simulink model "singledof_base"  (Simulink 7.8)
settings: Solver=FixedStepDiscrete  StartTime=0.0  StopTime=inf  FixedStep=Ts  RelTol=1e-3
PreLoadFcn:
  | loadParametersSingleDof
InitFcn:
  | loadParametersSingleDof
values from neighbouring files (symbols this model uses):
  L_arm = 0.075    [freemot.mat]    (also in loadParametersSingleDof.m)
  lowOrder_tfd_foh = c2d(tf([1 2*pi*.64154],[1 0]),Ts,'foh')    [loadParametersSingleDof.m]
  maxTorque_allowed = 1.125    [freemot.mat]    (also in loadParametersSingleDof.m)
  torque_constant = 3.112    [freemot.mat]    (also in loadParametersSingleDof.m)
  Ts = 0.0005    [freemot.mat]
undefined symbols (not defined in the file or in its folder): DiscIntNeverNeededParam, shuntDynPredict_part1_tfd_foh, shuntDynPredict_part2_tfd_foh
libraries: simulink x30, simulink_extras x3
(part 1 of 2)
settings Model: Creator=root  LastModifiedBy=root  SimulationMode=external  ExtModeTrigDuration=10000  ExtModeAutoUpdateStatusClock=off
settings OptimizationCC: InitFltsAndDblsToZero=on
settings DebuggingCC: SaveWithParameterizedLinksMsg=none  SignalResolutionControl=TryResolveAllWithWarning  MultiTaskDSMMsg=warning  MultiTaskCondExecSysMsg=none  FcnCallInpInsideContextMsg=Use local settings  StrictBusMsg=None
settings RTWCC: SystemTargetFile=ectarget.tlc  MakeCommand=make_rtw OPTS='-DNETIF_ID=1'  TemplateMakefile=ec_unix.tmf  Description=Ethercattarget Real-Time Target for PREEMPT-RT/Linux  ProcessScript=ectarget_make_rtw_hook  IncludeERTFirstTime=on
settings GRTTargetCC: TargetFcnLib=ansi_tfl_tmw.mat  ExtMode=on

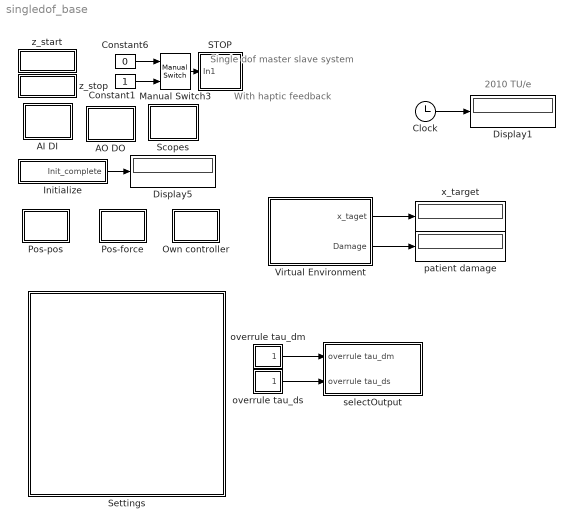
== system singledof_base ==
  note: With haptic feedback
  note: 2010 TU/e
  note: Single dof master slave system
  AI DI : Subsystem
      mask Display: disp('AI / DI')
  AO DO : Subsystem
      mask Display: disp('AO / DO')
  Clock : Clock
  Constant1 : Constant
  Constant6 : Constant  Value=0
  Display1 : Display
      settings: Decimation=200
  Display5 : Display
      settings: Decimation=200
  Initialize : Subsystem
  Manual Switch3 : simulink/Signal Routing/Manual Switch  sw=1  action=0  varsize=off
  Own controller : Subsystem
  Pos-force : Subsystem  mask{Ps=8, Is=0, Ds=0.1, bw_mode=off, fc=20, useI=on}
      mask prompts: Ps "Proportional action Position Slave"; Is "Integral action Position Slave"; Ds "Differential action Position Slave"; bw_mode "Or enter bandwidth:"; fc "Enter bandwidth (Hz) (max 70Hz)"; useI "Use Integral action"
      mask CallbackString:
      | |||temp=get_param(gcb,'bw_mode');
      | 
      | if(strcmp(temp,'off'))
      |    set_param(gcb,'MaskEnables',{'on','on','on','on','off','off'})
      | else
      |        set_param(gcb,'MaskEnables',{'off','off','off','on','on','on'})
      | end|
      | if strcmp(get_param(gcb,'bw_mode'),'on')
      |     wc=2*pi*eval(get_param(gcb,'fc'));
      |     if strcmp(get_param(gcb,'useI'),'on')
      |         C_tf=tf([1/wc 1 wc/5],[1 0]);
      |     else
      |         C_tf=tf([1/wc 1],1);
      |     end
      |     C_tf=minreal(C_tf/abs(freqresp(C_tf*fit_g22_s_2,wc)));
      |     set_param(gcb,'Ds',num2str(C_tf.num{1}(1)));
      |     set_param(gcb,'Ps',num2str(C_tf.num{1}(2)));
      | 
      |     if strcmp(get_param(gcb,'useI'),'on')
      |         set_param(gcb,'Is',num2str(C_tf.num{1}(3)));
      |     else
      |         set_param(gcb,'Is','0');
      |     end
      | end|temp=get_param(gcb,'maskCallbacks');
      | eval(temp{5})
  Pos-pos : Subsystem  mask{Pm=15, Im=0, Dm=.1, bw_modem=off, fcm=20, useIm=off, Ps=15, Is=0, Ds=.1, bw_modes=off, fcs=20, useIs=off}
      mask prompts: Pm "Proportional action master"; Im "Integral action master"; Dm "Differential action master"; bw_modem "Or enter bandwidth"; fcm "Bandwidth (Hz) (max 70Hz)"; useIm "Use Integral action"; Ps "Proportional action slave"; Is "Integral action slave"; Ds "Differential action slave"; bw_modes "Or enter bandwidth"; fcs "Bandwidth (Hz) (max 70Hz)"; useIs "Use Integral action"
      mask CallbackString:
      | |||temp=get_param(gcb,'bw_modem');
      | temps=get_param(gcb,'bw_modes');
      | 
      | if strcmp(temp,'off') & strcmp(temps,'off')
      |    set_param(gcb,'MaskEnables',{'on','on','on','on','off','off','on','on','on','on','off','off'})
      | elseif strcmp(temp,'on') & strcmp(temps,'off')
      |    set_param(gcb,'MaskEnables',{'off','off','off','on','on','on','on','on','on','on','off','off'})
      | elseif strcmp(temp,'off') & strcmp(temps,'on')
      |    set_param(gcb,'MaskEnables',{'on','on','on','on','off','off','off','off','off','on','on','on'})
      | else
      |    set_param(gcb,'MaskEnables',{'off','off','off','on','on','on','off','off','off','on','on','on'})
      | end|if strcmp(get_param(gcb,'bw_modem'),'on')
      |     wc=2*pi*eval(get_param(gcb,'fcm'));
      |     if strcmp(get_param(gcb,'useIm'),'on')
      |         C_tf=tf([1/wc 1 wc/5],[1 0]);
      |     else
      |         C_tf=tf([1/wc 1],1);
      |     end
      |     C_tf=minreal(C_tf/abs(freqresp(C_tf*fit_g22_m_2,wc)));
      |     set_param(gcb,'Dm',num2str(C_tf.num{1}(1)));
      |     set_param(gcb,'Pm',num2str(C_tf.num{1}(2)));
      | 
      |     if strcmp(get_param(gcb,'useIm'),'on')
      |         set_param(gcb,'Im',num2str(C_tf.num{1}(3)));
      |     else
      |         set_param(gcb,'Im','0');
      |     end
      | end|temp=get_param(gcb,'maskCallbacks');
      | eval(temp{5})||||temp=get_param(gcb,'maskCallbacks');
      | eval(temp{4})|if strcmp(get_param(gcb,'bw_modes'),'on')
      |     wc=2*pi*eval(get_param(gcb,'fcs'));
      |     if strcmp(get_param(gcb,'useIs'),'on')
      |         C_tf=tf([1/wc 1 wc/5],[1 0]);
      |     else
      |         C_tf=tf([1/wc 1],1);
      |     end
      |     C_tf=minreal(C_tf/abs(freqresp(C_tf*fit_g22_s_2,wc)));
      |     set_param(gcb,'Ds',num2str(C_tf.num{1}(1)));
      |     set_param(gcb,'Ps',num2str(C_tf.num{1}(2)));
      | 
      |     if strcmp(get_param(gcb,'useIs'),'on')
      |         set_param(gcb,'Is',num2str(C_tf.num{1}(3)));
      |     else
      |         set_param(gcb,'Is','0');
      |     end
      | end|temp=get_param(gcb,'maskCallbacks');
      | eval(temp{11})
  STOP : Subsystem
  Scopes : Subsystem
      mask Display: disp('Scopes')
  Settings : Subsystem  mask{mode=Own-controller, mu=1, lambda=1, comm_delay=0}
      mask prompts: mode "Control algorithm"; mu "Position scaling (mu)"; lambda "Force scaling (lambda)"; comm_delay "Communication delay"
      mask init:
      | bn{1}='off';
      | bn{2}='on';
      mask StyleString: popup(Position-position|Position-force|Own-controller|Overrule),edit,edit,edit
      mask Display:
      | text(.05,15/16,['Active mode: ' get_param(gcb,'mode')])
      | 
      | text(.05,13/16,['Position scaling (mu): ' num2str(mu)])
      | text(.05,12/16,['Force scaling (lambda): ' num2str(lambda)])
      | 
      | text(.05,10/16,['Communication delay: ' num2str(comm_delay) ' s'])
  Virtual Environment : Subsystem
  overrule tau_dm : Subsystem  LoadFcn=slideg Load  StartFcn=slideg StartFcn  StopFcn=slideg StopFcn  mask(Slider Gain){low=0, gain=0, high=0.5}
      settings: CopyFcn=slideg Copy  DeleteFcn=slideg DeleteBlock  NameChangeFcn=slideg NameChange  OpenFcn=slideg Open  CloseFcn=slideg Close  ParentCloseFcn=slideg ParentClose
      mask Display: disp(gain)
  overrule tau_ds : Subsystem  LoadFcn=slideg Load  StartFcn=slideg StartFcn  StopFcn=slideg StopFcn  mask(Slider Gain){low=0, gain=0, high=0.5}
      settings: CopyFcn=slideg Copy  DeleteFcn=slideg DeleteBlock  NameChangeFcn=slideg NameChange  OpenFcn=slideg Open  CloseFcn=slideg Close  ParentCloseFcn=slideg ParentClose
      mask Display: disp(gain)
  patient damage : Display
  selectOutput : Subsystem
  x_target : Display
  z_start : Subsystem
      settings: OpenFcn=|
      | set_param(bdroot(gcs),'SimulationCommand','connect')
      | set_param(bdroot(gcs),'SimulationCommand','start')
      mask Display: disp('start')
  z_stop : Subsystem
      settings: OpenFcn=set_param('singledof_demo/Initialize/ShutdownSim','Value',int2str(eval(get_param('singledof_demo/Initialize/ShutdownSim','Value'))+1))
      mask Display: disp('stop')
  wires:
  Initialize/1(Init_complete) -> Display5/1
  Clock/1 -> Display1/1
  Manual Switch3/1 -> STOP/1(In1)
  Constant6/1 -> Manual Switch3/1
  Constant1/1 -> Manual Switch3/2
  overrule tau_dm/1(Out1) -> selectOutput/1(overrule tau_dm)
  overrule tau_ds/1(Out1) -> selectOutput/2(overrule tau_ds)
  Virtual Environment/1(x_taget) -> x_target/1
  Virtual Environment/2(Damage) -> patient damage/1

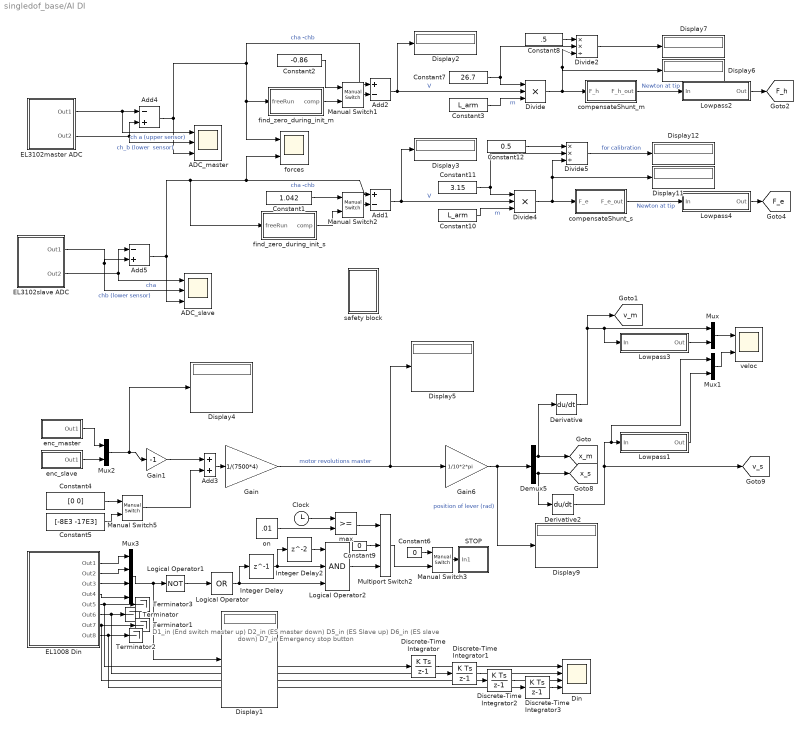
== system singledof_base/AI DI ==
  note: D1_in (End switch master up)
      | D2_in (ES master down)
      | D5_in (ES Slave up)
      | D6_in (ES slave down)
      | D7_in Emergency stop button
  ADC_master : Scope  NumInputPorts=3
      settings: TimeRange=5  YMin=7.605~1.4075~-6.204  YMax=7.6275~1.43~-6.192  SaveName=env_est2  MaxDataPoints=10000
  ADC_slave : Scope  NumInputPorts=3
      settings: TimeRange=5  YMin=2.775~-5~-7.5  YMax=2.975~10~7.5  SaveName=env_est3  MaxDataPoints=10000
  Add1 : Sum  Inputs=+-
  Add2 : Sum  Inputs=+-
  Add3 : Sum
  Add4 : Sum  Inputs=-+
  Add5 : Sum  Inputs=-+
  Clock : Clock
  Constant1 : Constant  Value=1.042
  Constant10 : Constant  Value=L_arm
  Constant11 : Constant  Value=3.15
  Constant12 : Constant  Value=0.5
  Constant2 : Constant  Value=-0.86
  Constant3 : Constant  Value=L_arm
  Constant4 : Constant  Value=[0 0]
  Constant5 : Constant  Value=[-8E3 -17E3]
  Constant6 : Constant  Value=0
  Constant7 : Constant  Value=26.7
  Constant8 : Constant  Value=.5
  Constant9 : Constant  Value=0
  Demux5 : Demux  Outputs=2
  Derivative : Derivative
  Derivative2 : Derivative
  Din : Scope  NumInputPorts=4
      settings: TimeRange=5  YMin=-5~-5~-5~-5  YMax=10~10~5~5  SaveName=env_est5  MaxDataPoints=10000
  Discrete-Time Integrator{,1..3} (4 alike) : DiscreteIntegrator  SampleTime=Ts  ICPrevOutput=DiscIntNeverNeededParam  ICPrevScaledInput=DiscIntNeverNeededParam
  Display{1..7,9,11..12} (10 alike) : Display
      settings: Decimation=200
  Divide : Product  Inputs=***
  Divide2 : Product  Inputs=**/
  Divide4 : Product  Inputs=***
  Divide5 : Product  Inputs=**/
  EL1008 Din : Subsystem  mask(EL1008){link_id=0}
      mask prompts: link_id "Link id (>=0)"
  EL3102master ADC : Subsystem  mask(EL3102){link_id=0}
      mask prompts: link_id "Link id (>=0)"
  EL3102slave ADC : Subsystem  mask(EL3102){link_id=1}
      mask prompts: link_id "Link id (>=0)"
  Gain : Gain  Gain=1/(7500*4)
  Gain1 : Gain  Gain=-1
  Gain6 : Gain  Gain=1/10*2*pi
  Integer Delay : Delay  DelayLength=1
  Integer Delay2 : Delay
  Logical Operator : Logic  Operator=OR  Inputs=1  AllPortsSameDT=off  OutDataTypeStr=boolean
  Logical Operator1 : Logic  Operator=NOT  Inputs=1  AllPortsSameDT=off  OutDataTypeStr=boolean
  Logical Operator2 : Logic  Inputs=3  AllPortsSameDT=off  OutDataTypeStr=boolean
  Lowpass1 : Subsystem  mask{cf=100}
      mask prompts: cf "Cut off Frequency"
      mask help:
      | Discrete time first order lowpass filter, with cut-off frequency cf (Hz)
      | Kz / (z+K-1), with K=2*pi*cf*TS
      | For low frequencies this corresponds to the continous time lowpass filter
      | tf(1,[1/(2*pi*cf) 1])
      |
      | The maximum value for K=1, in this case output equals input
      | e.g. for 4000Hz sampling frequency the maximum value cf=4000/(2*pi)=637Hz.
      mask Display: text(.1,.5,['Lowpass @' num2str(cf) 'Hz'])
  Lowpass2 : Subsystem  mask{cf=40}
      mask prompts: cf "Cut off Frequency"
      mask help:
      | Discrete time first order lowpass filter, with cut-off frequency cf (Hz)
      | Kz / (z+K-1), with K=2*pi*cf*TS
      | For low frequencies this corresponds to the continous time lowpass filter
      | tf(1,[1/(2*pi*cf) 1])
      |
      | The maximum value for K=1, in this case output equals input
      | e.g. for 4000Hz sampling frequency the maximum value cf=4000/(2*pi)=637Hz.
      mask Display: text(.1,.5,['Lowpass @' num2str(cf) 'Hz'])
  Lowpass3 : Subsystem  mask{cf=100}
      mask prompts: cf "Cut off Frequency"
      mask help:
      | Discrete time first order lowpass filter, with cut-off frequency cf (Hz)
      | Kz / (z+K-1), with K=2*pi*cf*TS
      | For low frequencies this corresponds to the continous time lowpass filter
      | tf(1,[1/(2*pi*cf) 1])
      |
      | The maximum value for K=1, in this case output equals input
      | e.g. for 4000Hz sampling frequency the maximum value cf=4000/(2*pi)=637Hz.
      mask Display: text(.1,.5,['Lowpass @' num2str(cf) 'Hz'])
  Lowpass4 : Subsystem  mask{cf=40}
      mask prompts: cf "Cut off Frequency"
      mask help:
      | Discrete time first order lowpass filter, with cut-off frequency cf (Hz)
      | Kz / (z+K-1), with K=2*pi*cf*TS
      | For low frequencies this corresponds to the continous time lowpass filter
      | tf(1,[1/(2*pi*cf) 1])
      |
      | The maximum value for K=1, in this case output equals input
      | e.g. for 4000Hz sampling frequency the maximum value cf=4000/(2*pi)=637Hz.
      mask Display: text(.1,.5,['Lowpass @' num2str(cf) 'Hz'])
  Manual Switch1 : simulink/Signal Routing/Manual Switch  sw=0  action=0  varsize=off
  Manual Switch2 : simulink/Signal Routing/Manual Switch  sw=0  action=0  varsize=off
  Manual Switch3 : simulink/Signal Routing/Manual Switch  sw=1  action=0  varsize=off
  Manual Switch5 : simulink/Signal Routing/Manual Switch  sw=1  action=0  varsize=off
  Multiport Switch2 : MultiPortSwitch  DataPortOrder=Zero-based contiguous  Inputs=2  zeroidx=on
  Mux : Mux  Inputs=2
  Mux1 : Mux  Inputs=2
  Mux2 : Mux  Inputs=2
  Mux3 : Mux
  STOP : Subsystem
  Terminator{,1..3} (4 alike) : Terminator
  compensateShunt_m : Subsystem
  compensateShunt_s : Subsystem
  enc_master : Subsystem
  enc_slave : Subsystem
  find_zero_during_init_m : Subsystem
  find_zero_during_init_s : Subsystem
  forces : Scope  NumInputPorts=2
      settings: TimeRange=6.25  YMin=-1.275~7.5  YMax=-0.95~9.4  SaveName=env_est4  MaxDataPoints=10000
  max : RelationalOperator  DisableCoverage=on
  on : Constant  DisableCoverage=on  Value=.01
  safety block : Subsystem
  veloc : Scope  NumInputPorts=2
      settings: TimeRange=6.25  YMin=-40000~-40000  YMax=40000~40000  SaveName=env_est1  MaxDataPoints=10000
  tag scope: F_e=global, F_h=global, v_m=global, v_s=global, x_m=global, x_s=global
  wires:
  Gain/1 -> Gain6/1, Display5/1  "motor revolutions master"
  Mux2/1 -> Gain1/1, Display4/1
  Add3/1 -> Gain/1
  Gain1/1 -> Add3/1
  Mux3/1 -> Display1/1, Logical Operator1/1
  Gain6/1 -> Demux5/1, Display9/1  "position of lever (rad)"
  Demux5/1 -> Derivative/1, [x_m]
  Demux5/2 -> Derivative2/1, [x_s]
  Derivative/1 -> Mux/1, Lowpass3/1(In), [v_m]
  Derivative2/1 -> Mux1/1, Lowpass1/1(In), [v_s]
  Logical Operator/1 -> Integer Delay/1, Logical Operator2/3
  Manual Switch3/1 -> STOP/1(In1)
  Constant6/1 -> Manual Switch3/1
  Integer Delay2/1 -> Logical Operator2/1
  Mux/1 -> veloc/1
  Mux1/1 -> veloc/2
  Lowpass3/1(Out) -> Mux/2
  Lowpass1/1(Out) -> Mux1/2
  EL1008 Din/1(Out1) -> Mux3/1
  EL1008 Din/2(Out2) -> Mux3/2
  EL1008 Din/3(Out3) -> Mux3/3
  EL1008 Din/4(Out4) -> Mux3/4
  EL1008 Din/7(Out7) -> Terminator1/1, Discrete-Time Integrator2/1
  EL1008 Din/8(Out8) -> Terminator2/1, Discrete-Time Integrator3/1
  EL1008 Din/5(Out5) -> Terminator3/1, Discrete-Time Integrator/1
  Logical Operator1/1 -> Logical Operator/1
  Integer Delay/1 -> Integer Delay2/1, Logical Operator2/2
  Constant4/1 -> Manual Switch5/1
  Constant5/1 -> Manual Switch5/2
  Manual Switch5/1 -> Add3/2
  Multiport Switch2/1 -> Manual Switch3/2
  Logical Operator2/1 -> Multiport Switch2/3
  Constant9/1 -> Multiport Switch2/2
  max/1 -> Multiport Switch2/1
  on/1 -> max/2
  Clock/1 -> max/1
  EL1008 Din/6(Out6) -> Terminator/1, Discrete-Time Integrator1/1
  Discrete-Time Integrator/1 -> Din/1
  Discrete-Time Integrator1/1 -> Din/2
  Discrete-Time Integrator2/1 -> Din/3
  Discrete-Time Integrator3/1 -> Din/4
  enc_master/1(Out1) -> Mux2/1
  enc_slave/1(Out1) -> Mux2/2
  Add2/1 -> Display2/1, Divide/2  "V"
  Manual Switch1/1 -> Add2/2
  Constant2/1 -> Manual Switch1/1
  find_zero_during_init_m/1(comp) -> Manual Switch1/2
  Divide/1 -> Display6/1, Divide2/3, compensateShunt_m/1(F_h)
  compensateShunt_m/1(F_h_out) -> Lowpass2/1(In)  "Newton at tip"
  Constant3/1 -> Divide/3  "m"
  Constant7/1 -> Divide/1, Divide2/2
  Add1/1 -> Divide4/2, Display3/1  "V"
  Manual Switch2/1 -> Add1/2
  Constant1/1 -> Manual Switch2/1
  find_zero_during_init_s/1(comp) -> Manual Switch2/2
  compensateShunt_s/1(F_e_out) -> Lowpass4/1(In)  "Newton at tip"
  Divide4/1 -> compensateShunt_s/1(F_e), Display11/1, Divide5/3
  Constant10/1 -> Divide4/3  "m"
  Constant11/1 -> Divide4/1, Divide5/2
  Constant12/1 -> Divide5/1
  Divide5/1 -> Display12/1  "for calibration"
  Lowpass2/1(Out) -> [F_h]
  Lowpass4/1(Out) -> [F_e]
  Divide2/1 -> Display7/1
  Constant8/1 -> Divide2/1
  EL3102master ADC/1(Out1) -> Add4/1, ADC_master/1  "ch a (upper sensor)"
  EL3102master ADC/2(Out2) -> ADC_master/2, Add4/2  "ch_b (lower  sensor)"
  Add4/1 -> forces/1, find_zero_during_init_m/1(freeRun), Add2/1, ADC_master/3  "cha -chb"
  EL3102slave ADC/1(Out1) -> ADC_slave/2, Add5/2  "chb (lower sensor)"
  EL3102slave ADC/2(Out2) -> ADC_slave/1, Add5/1  "cha"
  Add5/1 -> Add1/1, forces/2, find_zero_during_init_s/1(freeRun), ADC_slave/3  "cha -chb"

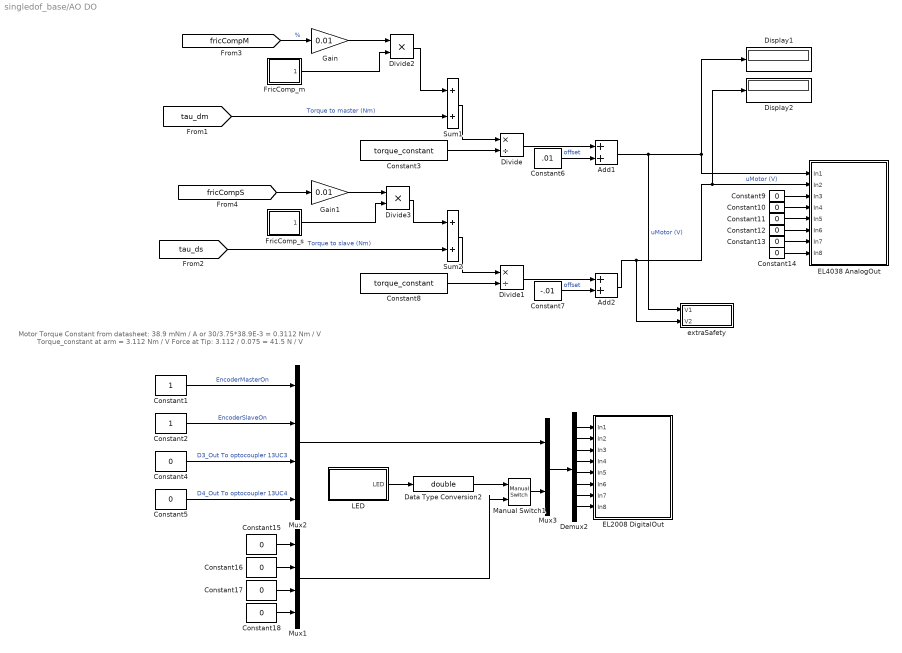
== system singledof_base/AO DO ==
  note: Motor Torque Constant from datasheet: 38.9 mNm / A or 30/3.75*38.9E-3 = 0.3112 Nm / V
      | Torque_constant at arm = 3.112 Nm / V
      | Force at Tip: 3.112 / 0.075 = 41.5 N / V
  Add1 : Sum
  Add2 : Sum
  Constant1 : Constant
  Constant{4..5,9..18} (12 alike) : Constant  Value=0
  Constant2 : Constant
  Constant3 : Constant  Value=torque_constant
  Constant6 : Constant  Value=.01
  Constant7 : Constant  Value=-.01
  Constant8 : Constant  Value=torque_constant
  Data Type Conversion2 : DataTypeConversion  OutDataTypeStr=double
  Demux2 : Demux  Outputs=8
  Display1 : Display
      settings: Decimation=200
  Display2 : Display
      settings: Decimation=200
  Divide : Product  Inputs=*/
  Divide1 : Product  Inputs=*/
  Divide2 : Product  Inputs=**
  Divide3 : Product  Inputs=**
  EL2008 DigitalOut : Subsystem  mask(EL2008){link_id=0}
      mask prompts: link_id "Link id (>=0)"
  EL4038 AnalogOut : Subsystem  mask(EL4038){link_id=0}
      mask prompts: link_id "Link id (>=0)"
  FricComp_m : Subsystem
      mask Display: plot([-1 0 0 1],[-1-2, -1, 1, 1+2], [-1 1],[0 0],[0 0],[-3,3])
  FricComp_s : Subsystem
      mask Display: plot([-1 0 0 1],[-1-2, -1, 1, 1+2], [-1 1],[0 0],[0 0],[-3,3])
  Gain : Gain  Gain=0.01
  Gain1 : Gain  Gain=0.01
  LED : Subsystem
  Manual Switch1 : simulink/Signal Routing/Manual Switch  sw=0  action=0  varsize=off
  Mux1 : Mux
  Mux2 : Mux
  Mux3 : Mux  Inputs=2
  Sum1 : Sum
  Sum2 : Sum
  extraSafety : Subsystem
  wires:
  Demux2/8 -> EL2008 DigitalOut/8(In8)
  Demux2/7 -> EL2008 DigitalOut/7(In7)
  Demux2/6 -> EL2008 DigitalOut/6(In6)
  Demux2/5 -> EL2008 DigitalOut/5(In5)
  Demux2/4 -> EL2008 DigitalOut/4(In4)
  Demux2/3 -> EL2008 DigitalOut/3(In3)
  Demux2/2 -> EL2008 DigitalOut/2(In2)
  Demux2/1 -> EL2008 DigitalOut/1(In1)
  Constant14/1 -> EL4038 AnalogOut/8(In8)
  Constant13/1 -> EL4038 AnalogOut/7(In7)
  Constant12/1 -> EL4038 AnalogOut/6(In6)
  Constant11/1 -> EL4038 AnalogOut/5(In5)
  Constant10/1 -> EL4038 AnalogOut/4(In4)
  Constant9/1 -> EL4038 AnalogOut/3(In3)
  [fricCompS] -> Gain1/1
  Gain/1 -> Divide2/1
  Divide2/1 -> Sum1/1
  Gain1/1 -> Divide3/1
  Divide3/1 -> Sum2/1
  [fricCompM] -> Gain/1  "%"
  FricComp_s/1(FricCompOut) -> Divide3/2
  FricComp_m/1(FricCompOut) -> Divide2/2
  Sum2/1 -> Divide1/1
  Sum1/1 -> Divide/1
  Mux3/1 -> Demux2/1
  LED/1(LED) -> Data Type Conversion2/1
  Mux2/1 -> Mux3/1
  [tau_ds] -> Sum2/2  "Torque to slave (Nm)"
  [tau_dm] -> Sum1/2  "Torque to master (Nm)"
  Constant8/1 -> Divide1/2
  Constant3/1 -> Divide/2
  Divide1/1 -> Add2/1
  Divide/1 -> Add1/1
  Constant7/1 -> Add2/2  "offset"
  Add2/1 -> Display2/1, EL4038 AnalogOut/2(In2), extraSafety/2(V2)  "uMotor (V)"
  Constant6/1 -> Add1/2  "offset"
  Add1/1 -> Display1/1, EL4038 AnalogOut/1(In1), extraSafety/1(V1)  "uMotor (V)"
  Constant5/1 -> Mux2/4  "D4_Out To optocoupler 13UC4"
  Constant4/1 -> Mux2/3  "D3_Out To optocoupler 13UC3"
  Constant2/1 -> Mux2/2  "EncoderSlaveOn"
  Constant1/1 -> Mux2/1  "EncoderMasterOn"
  Constant15/1 -> Mux1/1
  Constant16/1 -> Mux1/2
  Constant17/1 -> Mux1/3
  Constant18/1 -> Mux1/4
  Manual Switch1/1 -> Mux3/2
  Mux1/1 -> Manual Switch1/2
  Data Type Conversion2/1 -> Manual Switch1/1

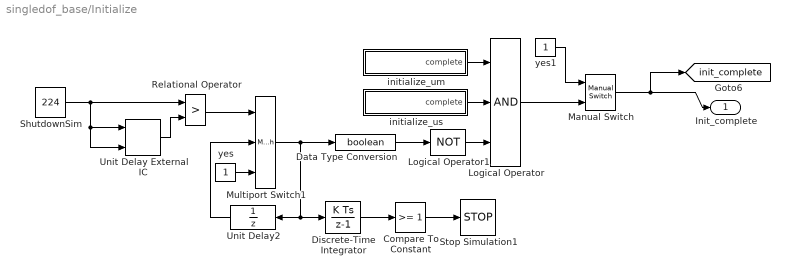
== system singledof_base/Initialize ==
  Compare To Constant : simulink/Logic and Bit Operations/Compare To Constant  relop=>=  const=1  OutDataTypeStr=boolean
  Data Type Conversion : DataTypeConversion  OutDataTypeStr=boolean
  Discrete-Time Integrator : DiscreteIntegrator  SampleTime=Ts  ICPrevOutput=DiscIntNeverNeededParam  ICPrevScaledInput=DiscIntNeverNeededParam
  Logical Operator : Logic  Inputs=3  AllPortsSameDT=off  OutDataTypeStr=boolean
  Logical Operator1 : Logic  Operator=NOT  Inputs=3  AllPortsSameDT=off  OutDataTypeStr=boolean
  Manual Switch : simulink/Signal Routing/Manual Switch  sw=1  action=0  varsize=off
  Multiport Switch1 : MultiPortSwitch  DataPortOrder=Zero-based contiguous  Inputs=2  zeroidx=on
  Relational Operator : RelationalOperator  Operator=>  OutDataTypeStr=boolean
  ShutdownSim : Constant  Value=224
  Stop Simulation1 : Stop
  Unit Delay External IC : simulink/Additional Math & Discrete/Additional Discrete/Unit Delay External IC  tsamp=-1
  Unit Delay2 : UnitDelay  SampleTime=-1
  initialize_um : Subsystem
  initialize_us : Subsystem
  yes : Constant
  yes1 : Constant
  Init_complete : Outport
  tag scope: init_complete=global
  wires:
  Manual Switch/1 -> Init_complete/1, [init_complete]
  Unit Delay External IC/1 -> Relational Operator/2
  ShutdownSim/1 -> Unit Delay External IC/2, Unit Delay External IC/1, Relational Operator/1
  Relational Operator/1 -> Multiport Switch1/1
  Compare To Constant/1 -> Stop Simulation1/1
  Discrete-Time Integrator/1 -> Compare To Constant/1
  Data Type Conversion/1 -> Logical Operator1/1
  Logical Operator1/1 -> Logical Operator/3
  yes/1 -> Multiport Switch1/3
  Unit Delay2/1 -> Multiport Switch1/2
  Multiport Switch1/1 -> Unit Delay2/1, Discrete-Time Integrator/1, Data Type Conversion/1
  initialize_um/1(complete) -> Logical Operator/1
  initialize_us/1(complete) -> Logical Operator/2
  Logical Operator/1 -> Manual Switch/2
  yes1/1 -> Manual Switch/1

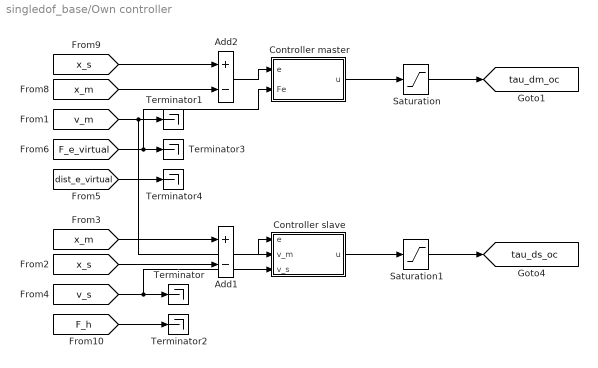
== system singledof_base/Own controller ==
  Add1 : Sum  Inputs=+-
  Add2 : Sum  Inputs=+-
  Controller master : Subsystem
      mask Display: text(.1,.5,'Controller')
  Controller slave : Subsystem
      mask Display: text(.1,.5,'Controller')
  Saturation : Saturate  UpperLimit=maxTorque_allowed  LowerLimit=-maxTorque_allowed
  Saturation1 : Saturate  UpperLimit=maxTorque_allowed  LowerLimit=-maxTorque_allowed
  Terminator{,1..4} (5 alike) : Terminator
  tag scope: tau_dm_oc=global, tau_ds_oc=global
  wires:
  [x_s] -> Add1/2
  Add1/1 -> Controller slave/1(e)
  Saturation/1 -> [tau_dm_oc]
  Saturation1/1 -> [tau_ds_oc]
  [x_m] -> Add1/1
  [x_m] -> Add2/2
  [x_s] -> Add2/1
  Add2/1 -> Controller master/1(e)
  [v_s] -> Terminator/1, Controller slave/3(v_s)
  [v_m] -> Terminator1/1, Controller slave/2(v_m)
  Controller master/1(u) -> Saturation/1
  Controller slave/1(u) -> Saturation1/1
  [F_h] -> Terminator2/1
  [F_e_virtual] -> Terminator3/1, Controller master/2(Fe)
  [dist_e_virtual] -> Terminator4/1

== system singledof_base/Pos-force ==
  Add1 : Sum  Inputs=+-
  Add2 : Sum  Inputs=+-
  Gain1 : Gain  Gain=-1
  Gain3 : Gain  Gain=0
  Product : Product  RndMeth=Zero
  Product1 : Product  RndMeth=Zero
  contr_s : Subsystem
      mask Display:
      | text(.1,.7,'Slave')
      | text(.1,.3,'Controller')
  master to slave : Subsystem
      mask Display: disp('Communication channel')
  slave to master : Subsystem
      mask Display: disp('Communication channel')
  tag scope: tau_dm_posforce=global, tau_ds_posforce=global
  wires:
  Gain1/1 -> Product1/1
  Gain3/1 -> Add2/2
  Add2/1 -> [tau_dm_posforce]
  [v_m] -> Gain3/1
  contr_s/1(u) -> [tau_ds_posforce]
  Product1/1 -> slave to master/1(In1)
  [F_e] -> Gain1/1
  [lambda] -> Product1/2
  slave to master/1(Out1) -> Add2/1
  master to slave/1(Out1) -> Add1/1
  Product/1 -> master to slave/1(In1)
  [x_m] -> Product/1
  [mu] -> Product/2
  [x_s] -> Add1/2
  Add1/1 -> contr_s/1(e)

== system singledof_base/Pos-pos ==
  Add1 : Sum  Inputs=+-
  Add2 : Sum  Inputs=+-
  Product : Product  RndMeth=Zero
  Product1 : Product  RndMeth=Zero
  contr_m : Subsystem
      mask Display: text(.1,.5,'Controller')
  contr_s : Subsystem
      mask Display: text(.1,.5,'Controller')
  master to slave : Subsystem
      mask Display: disp('Communication channel')
  slave to master : Subsystem
      mask Display: disp('Communication channel')
  tag scope: tau_dm_pospos=global, tau_ds_pospos=global
  wires:
  Product1/1 -> contr_m/1(e)
  Add2/1 -> Product1/1
  [lambda] -> Product1/2
  Add1/1 -> contr_s/1(e)
  [x_s] -> slave to master/1(In1), Add1/2
  master to slave/1(Out1) -> Add1/1
  Product/1 -> master to slave/1(In1), Add2/2
  [x_m] -> Product/1
  [mu] -> Product/2
  contr_m/1(u) -> [tau_dm_pospos]
  slave to master/1(Out1) -> Add2/1
  contr_s/1(u) -> [tau_ds_pospos]

== system singledof_base/STOP ==
  In1 : Inport
  Data Type Conversion : DataTypeConversion
  Data Type Conversion1 : DataTypeConversion
  Integer Delay1 : Delay  DelayLength=10
  S-R Flip-Flop : simulink_extras/Flip Flops/S-R Flip-Flop  initial_condition=0
  Stop Simulation1 : Stop
  Terminator4 : Terminator
  on2 : Constant  DisableCoverage=on  Value=0
  tag scope: settozero3=global
  wires:
  on2/1 -> Data Type Conversion/1
  Integer Delay1/1 -> Stop Simulation1/1
  S-R Flip-Flop/2 -> [settozero3]
  Data Type Conversion/1 -> S-R Flip-Flop/2
  In1/1 -> Data Type Conversion1/1
  S-R Flip-Flop/1 -> Terminator4/1
  Data Type Conversion1/1 -> S-R Flip-Flop/1, Integer Delay1/1

== system singledof_base/Scopes ==
  Gain2 : Gain  Gain=-1
  Gain3 : Gain  Gain=-1
  Mux2 : Mux  Inputs=2
  Mux3 : Mux  Inputs=2
  Mux4 : Mux  Inputs=2
  Scope : Scope  NumInputPorts=3
      settings: TimeRange=5  YMin=-0.4~-1~-1  YMax=0.7~2.5~1.25  SaveName=scope  MaxDataPoints=20000
  wires:
  Gain3/1 -> Mux4/1
  [F_h] -> Gain3/1
  [F_e] -> Mux4/2
  Gain2/1 -> Mux2/1
  Mux2/1 -> Scope/3  "Input torque (Nm at lever)      -tau_rm, tau_rs"
  [tau_dm] -> Gain2/1
  [tau_ds] -> Mux2/2
  Mux4/1 -> Scope/2  "Interaction forces (Nm at lever)     -F_h, F_e"
  [x_s] -> Mux3/2
  [x_m] -> Mux3/1
  Mux3/1 -> Scope/1  "Lever positions (rad) master, slave, wall"

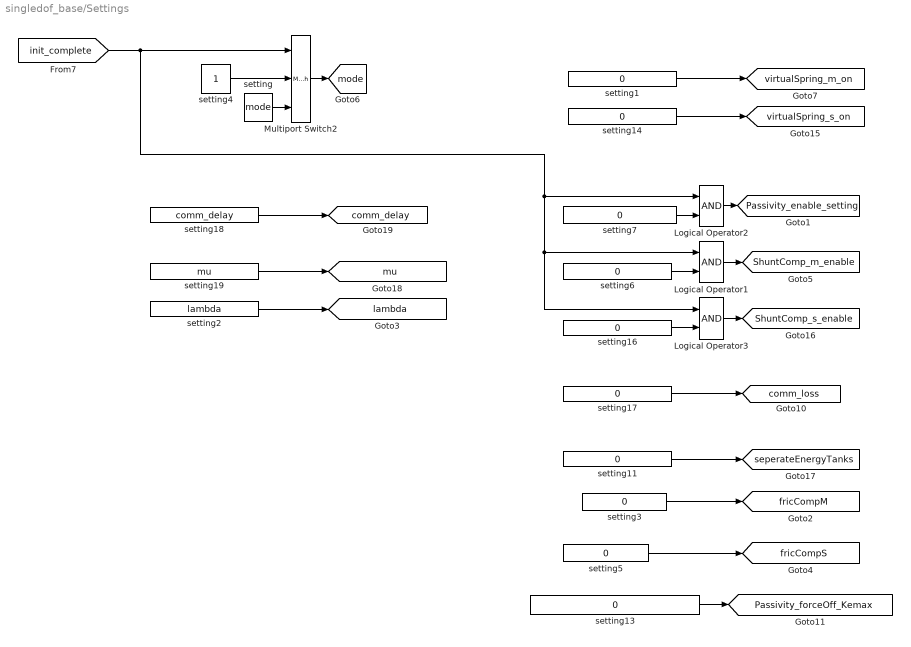
== system singledof_base/Settings ==
  Logical Operator1 : Logic  AllPortsSameDT=off  OutDataTypeStr=boolean
  Logical Operator2 : Logic  AllPortsSameDT=off  OutDataTypeStr=boolean
  Logical Operator3 : Logic  AllPortsSameDT=off  OutDataTypeStr=boolean
  Multiport Switch2 : MultiPortSwitch  DataPortOrder=Zero-based contiguous  Inputs=2  zeroidx=on
  setting : Constant  Value=mode
  setting{1,3,5..7,11,13..14,16..17} (10 alike) : Constant  Value=0
  setting18 : Constant  Value=comm_delay
  setting19 : Constant  Value=mu
  setting2 : Constant  Value=lambda
  setting4 : Constant
  tag scope: Passivity_enable_setting=global, Passivity_forceOff_Kemax=global, ShuntComp_m_enable=global, ShuntComp_s_enable=global, comm_delay=global, comm_loss=global, fricCompM=global, fricCompS=global, lambda=global, mode=global, mu=global, seperateEnergyTanks=global, virtualSpring_m_on=global, virtualSpring_s_on=global
  wires:
  [init_complete] -> Multiport Switch2/1, Logical Operator3/1, Logical Operator1/1, Logical Operator2/1
  Multiport Switch2/1 -> [mode]
  setting4/1 -> Multiport Switch2/2
  setting/1 -> Multiport Switch2/3
  setting13/1 -> [Passivity_forceOff_Kemax]
  setting11/1 -> [seperateEnergyTanks]
  setting5/1 -> [fricCompS]
  setting3/1 -> [fricCompM]
  setting2/1 -> [lambda]
  setting19/1 -> [mu]
  setting18/1 -> [comm_delay]
  setting17/1 -> [comm_loss]
  Logical Operator3/1 -> [ShuntComp_s_enable]
  setting16/1 -> Logical Operator3/2
  setting14/1 -> [virtualSpring_s_on]
  setting1/1 -> [virtualSpring_m_on]
  Logical Operator1/1 -> [ShuntComp_m_enable]
  setting6/1 -> Logical Operator1/2
  setting7/1 -> Logical Operator2/2
  Logical Operator2/1 -> [Passivity_enable_setting]

== system singledof_base/Virtual Environment ==
  Virtual Environment : S-Function  FunctionName=VirtualEnvironment_sf  EnableBusSupport=off
  x_taget : Outport
  Damage : Outport  Port=2
  tag scope: F_e_virtual=global, dist_e_virtual=global
  wires:
  [x_s] -> Virtual Environment/1
  [v_s] -> Virtual Environment/2
  [mode] -> Virtual Environment/3
  Virtual Environment/1 -> [F_e_virtual]
  Virtual Environment/2 -> x_taget/1
  Virtual Environment/3 -> Damage/1
  Virtual Environment/4 -> [dist_e_virtual]

== system singledof_base/overrule tau_dm ==
  Setpoint : Gain  Gain=gain  SaturateOnIntegerOverflow=on  OutDataTypeStr=Inherit: Same as input  ParamDataTypeStr=Inherit: Same as input
  constant : Constant
  Out1 : Outport
  wires:
  constant/1 -> Setpoint/1
  Setpoint/1 -> Out1/1

== system singledof_base/overrule tau_ds ==
  Setpoint : Gain  Gain=gain  SaturateOnIntegerOverflow=on  OutDataTypeStr=Inherit: Same as input  ParamDataTypeStr=Inherit: Same as input
  constant : Constant
  Out1 : Outport
  wires:
  Setpoint/1 -> Out1/1
  constant/1 -> Setpoint/1

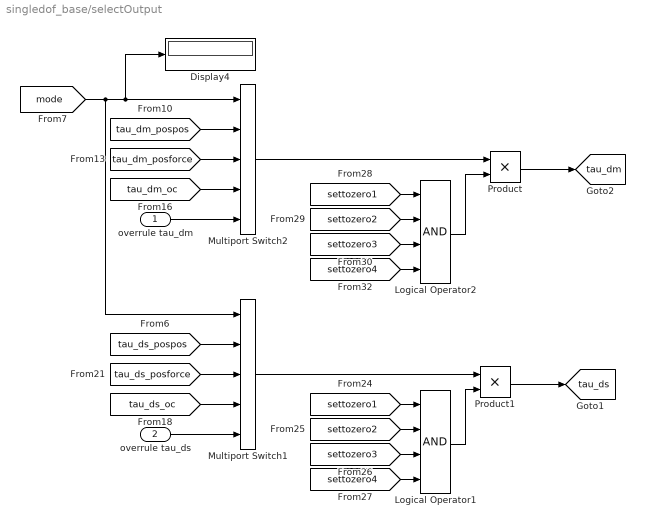
== system singledof_base/selectOutput ==
  overrule tau_dm : Inport
  overrule tau_ds : Inport  Port=2
  Display4 : Display
  Logical Operator1 : Logic  Inputs=4  AllPortsSameDT=off  OutDataTypeStr=boolean
  Logical Operator2 : Logic  Inputs=4  AllPortsSameDT=off  OutDataTypeStr=boolean
  Multiport Switch1 : MultiPortSwitch  Inputs=4  zeroidx=off
  Multiport Switch2 : MultiPortSwitch  Inputs=4  zeroidx=off
  Product : Product  RndMeth=Zero
  Product1 : Product  RndMeth=Zero
  tag scope: tau_dm=global, tau_ds=global
  wires:
  [tau_dm_pospos] -> Multiport Switch2/2
  [tau_dm_posforce] -> Multiport Switch2/3
  [mode] -> Multiport Switch2/1, Display4/1, Multiport Switch1/1
  Logical Operator2/1 -> Product/2
  Product/1 -> [tau_dm]
  Logical Operator1/1 -> Product1/2
  Product1/1 -> [tau_ds]
  [settozero1] -> Logical Operator2/1
  [settozero3] -> Logical Operator2/3
  [settozero4] -> Logical Operator2/4
  [settozero1] -> Logical Operator1/1
  [settozero2] -> Logical Operator1/2
  [settozero3] -> Logical Operator1/3
  [settozero4] -> Logical Operator1/4
  [settozero2] -> Logical Operator2/2
  [tau_dm_oc] -> Multiport Switch2/4
  Multiport Switch2/1 -> Product/1
  Multiport Switch1/1 -> Product1/1
  [tau_ds_pospos] -> Multiport Switch1/2
  [tau_ds_posforce] -> Multiport Switch1/3
  [tau_ds_oc] -> Multiport Switch1/4
  overrule tau_ds/1 -> Multiport Switch1/5
  overrule tau_dm/1 -> Multiport Switch2/5

== system singledof_base/z_start ==

== system singledof_base/z_stop ==

== system singledof_base/AI DI/EL1008 Din ==
  Demux : Demux  Outputs=8
  ec_EL1008_di : S-Function  FunctionName=ec_EL1008_di  Parameters=link_id  EnableBusSupport=off  mask{link_id=link_id}
      mask prompts: link_id "digital in id (start from 1)"
  Out1 : Outport
  Out2 : Outport  Port=2
  Out3 : Outport  Port=3
  Out4 : Outport  Port=4
  Out5 : Outport  Port=5
  Out6 : Outport  Port=6
  Out7 : Outport  Port=7
  Out8 : Outport  Port=8
  wires:
  ec_EL1008_di/1 -> Demux/1
  Demux/1 -> Out1/1
  Demux/2 -> Out2/1
  Demux/3 -> Out3/1
  Demux/4 -> Out4/1
  Demux/5 -> Out5/1
  Demux/6 -> Out6/1
  Demux/7 -> Out7/1
  Demux/8 -> Out8/1

== system singledof_base/AI DI/EL3102master ADC ==
  Demux : Demux  Outputs=2
  ec_EL3102_adc : S-Function  FunctionName=ec_EL3102_adc  Parameters=link_id  EnableBusSupport=off  mask{link_id=link_id}
      mask prompts: link_id "analog in id (start from 1)"
  Out1 : Outport
  Out2 : Outport  Port=2
  wires:
  ec_EL3102_adc/1 -> Demux/1
  Demux/1 -> Out1/1
  Demux/2 -> Out2/1

== system singledof_base/AI DI/EL3102slave ADC ==
  Demux : Demux  Outputs=2
  ec_EL3102_adc : S-Function  FunctionName=ec_EL3102_adc  Parameters=link_id  EnableBusSupport=off  mask{link_id=link_id}
      mask prompts: link_id "analog in id (start from 1)"
  Out1 : Outport
  Out2 : Outport  Port=2
  wires:
  Demux/2 -> Out2/1
  Demux/1 -> Out1/1
  ec_EL3102_adc/1 -> Demux/1

== system singledof_base/AI DI/Lowpass1 ==
  In : Inport
  Constant1 : Constant
  Cut-off freq (Hz) : Constant  Value=cf
  Weighted Sample Time Math1 : SampleTimeMath  TsampMathOp=*
  lowpass : MATLAB Function  TreatAsAtomicUnit=on
  Out : Outport
  wires:
  Weighted Sample Time Math1/1 -> lowpass/3(Ts)
  Constant1/1 -> Weighted Sample Time Math1/1
  In/1 -> lowpass/1(in)
  lowpass/1(out) -> Out/1
  Cut-off freq (Hz)/1 -> lowpass/2(cf)

== system singledof_base/AI DI/Lowpass2 ==
  In : Inport
  Constant1 : Constant
  Cut-off freq (Hz) : Constant  Value=cf
  Weighted Sample Time Math1 : SampleTimeMath  TsampMathOp=*
  lowpass : MATLAB Function  TreatAsAtomicUnit=on
  Out : Outport
  wires:
  Cut-off freq (Hz)/1 -> lowpass/2(cf)
  lowpass/1(out) -> Out/1
  In/1 -> lowpass/1(in)
  Constant1/1 -> Weighted Sample Time Math1/1
  Weighted Sample Time Math1/1 -> lowpass/3(Ts)

== system singledof_base/AI DI/Lowpass3 ==
  In : Inport
  Constant1 : Constant
  Cut-off freq (Hz) : Constant  Value=cf
  Weighted Sample Time Math1 : SampleTimeMath  TsampMathOp=*
  lowpass : MATLAB Function  TreatAsAtomicUnit=on
  Out : Outport
  wires:
  Cut-off freq (Hz)/1 -> lowpass/2(cf)
  lowpass/1(out) -> Out/1
  In/1 -> lowpass/1(in)
  Constant1/1 -> Weighted Sample Time Math1/1
  Weighted Sample Time Math1/1 -> lowpass/3(Ts)

== system singledof_base/AI DI/Lowpass4 ==
  In : Inport
  Constant1 : Constant
  Cut-off freq (Hz) : Constant  Value=cf
  Weighted Sample Time Math1 : SampleTimeMath  TsampMathOp=*
  lowpass : MATLAB Function  TreatAsAtomicUnit=on
  Out : Outport
  wires:
  Cut-off freq (Hz)/1 -> lowpass/2(cf)
  lowpass/1(out) -> Out/1
  In/1 -> lowpass/1(in)
  Constant1/1 -> Weighted Sample Time Math1/1
  Weighted Sample Time Math1/1 -> lowpass/3(Ts)

== system singledof_base/AI DI/STOP ==
  In1 : Inport
  Data Type Conversion : DataTypeConversion
  Data Type Conversion1 : DataTypeConversion
  Integer Delay1 : Delay  DelayLength=10
  S-R Flip-Flop : simulink_extras/Flip Flops/S-R Flip-Flop  initial_condition=0
  Stop Simulation1 : Stop
  Terminator4 : Terminator
  on2 : Constant  DisableCoverage=on  Value=0
  tag scope: settozero1=global
  wires:
  on2/1 -> Data Type Conversion/1
  Integer Delay1/1 -> Stop Simulation1/1
  S-R Flip-Flop/2 -> [settozero1]
  Data Type Conversion/1 -> S-R Flip-Flop/2
  In1/1 -> Data Type Conversion1/1
  S-R Flip-Flop/1 -> Terminator4/1
  Data Type Conversion1/1 -> S-R Flip-Flop/1, Integer Delay1/1

== system singledof_base/AI DI/compensateShunt_m ==
  F_h : Inport
  Add5 : Sum  Inputs=+-
  Constant1 : Constant  Value=1/2000*3
  Constant2 : Constant  Value=0
  Correction factor : Gain  Gain=1.05
  Discrete Transfer Fcn : DiscreteTransferFcn  Numerator=lowOrder_tfd_foh.num{1}  Denominator=lowOrder_tfd_foh.den{1}  SampleTime=Ts
  ForceSensor_actuatorTorque_comparison : Scope  NumInputPorts=2
      settings: TimeRange=6.25  YMin=-0.05~0.25  YMax=0.65~0.65  SaveName=scopeShunt  MaxDataPoints=20000
  Multiport Switch2 : MultiPortSwitch  DataPortOrder=Zero-based contiguous  Inputs=2  zeroidx=on
  Mux1 : Mux  Inputs=2
  Mux2 : Mux  Inputs=2
  ShuntDynPredicter Part 1 : DiscreteTransferFcn  Numerator=shuntDynPredict_part1_tfd_foh.num{1}  Denominator=shuntDynPredict_part1_tfd_foh.den{1}  SampleTime=Ts
  ShuntDynPredicter Part 2 : DiscreteTransferFcn  Numerator=shuntDynPredict_part2_tfd_foh.num{1}  Denominator=shuntDynPredict_part2_tfd_foh.den{1}  SampleTime=Ts
  TimeDelay1 : VariableTransportDelay  MaximumPoints=2000  FixedBuffer=on
  TimeDelay2 : VariableTransportDelay  MaximumPoints=2000  FixedBuffer=on
  F_h_out : Outport
  wires:
  Discrete Transfer Fcn/1 -> ShuntDynPredicter Part 2/1
  Constant2/1 -> TimeDelay1/2
  TimeDelay1/1 -> ShuntDynPredicter Part 1/1
  Mux1/1 -> ForceSensor_actuatorTorque_comparison/2
  Mux2/1 -> ForceSensor_actuatorTorque_comparison/1
  Constant1/1 -> TimeDelay2/2
  TimeDelay2/1 -> Discrete Transfer Fcn/1
  F_h/1 -> TimeDelay1/1, Mux1/1, Multiport Switch2/2
  ShuntDynPredicter Part 1/1 -> Mux2/1, Add5/1
  Add5/1 -> Mux1/2, Multiport Switch2/3
  Correction factor/1 -> Add5/2, Mux2/2
  [tau_rm] -> TimeDelay2/1
  ShuntDynPredicter Part 2/1 -> Correction factor/1
  Multiport Switch2/1 -> F_h_out/1
  [ShuntComp_m_enable] -> Multiport Switch2/1

== system singledof_base/AI DI/compensateShunt_s ==
  F_e : Inport
  Add5 : Sum  Inputs=+-
  Constant1 : Constant  Value=1/2000*3
  Constant2 : Constant  Value=0
  Correction factor : Gain  Gain=1.05
  Discrete Transfer Fcn : DiscreteTransferFcn  Numerator=lowOrder_tfd_foh.num{1}  Denominator=lowOrder_tfd_foh.den{1}  SampleTime=Ts
  Multiport Switch2 : MultiPortSwitch  DataPortOrder=Zero-based contiguous  Inputs=2  zeroidx=on
  ShuntDynPredicter Part 1 : DiscreteTransferFcn  Numerator=shuntDynPredict_part1_tfd_foh.num{1}  Denominator=shuntDynPredict_part1_tfd_foh.den{1}  SampleTime=Ts
  ShuntDynPredicter Part 2 : DiscreteTransferFcn  Numerator=shuntDynPredict_part2_tfd_foh.num{1}  Denominator=shuntDynPredict_part2_tfd_foh.den{1}  SampleTime=Ts
  TimeDelay1 : VariableTransportDelay  MaximumPoints=2000  FixedBuffer=on
  TimeDelay2 : VariableTransportDelay  MaximumPoints=2000  FixedBuffer=on
  F_e_out : Outport
  wires:
  Discrete Transfer Fcn/1 -> ShuntDynPredicter Part 2/1
  Constant2/1 -> TimeDelay1/2
  TimeDelay1/1 -> ShuntDynPredicter Part 1/1
  Constant1/1 -> TimeDelay2/2
  TimeDelay2/1 -> Discrete Transfer Fcn/1
  F_e/1 -> TimeDelay1/1, Multiport Switch2/2  "Unfiltered"
  Add5/1 -> Multiport Switch2/3  "Filtered"
  Correction factor/1 -> Add5/2
  [tau_rs] -> TimeDelay2/1
  Multiport Switch2/1 -> F_e_out/1
  [ShuntComp_s_enable] -> Multiport Switch2/1
  ShuntDynPredicter Part 1/1 -> Add5/1
  ShuntDynPredicter Part 2/1 -> Correction factor/1

== system singledof_base/AI DI/enc_master ==
  Add1 : Sum
  Add6 : Sum
  Constant4 : Constant  Value=18
  Display1 : Display
  Display2 : Display
  Display4 : Display
      settings: Decimation=200
  EL5101 Encoder : Subsystem  mask(EL5101){link_id=1}
      mask prompts: link_id "Link id (>=0)"
  EL5101 Latch : Subsystem  mask(EL5101){link_id=1}
      mask prompts: link_id "Link id (>=0)"
  Gain : Gain  Gain=1/(7500*4)
  Gain1 : Gain  Gain=-1
  Gain6 : Gain  Gain=1/10*360
  Out1 : Outport
  wires:
  EL5101 Encoder/1(Out1) -> Display4/1, Add6/1, Out1/1
  EL5101 Latch/1(Out1) -> Display1/1, Gain1/1
  Gain/1 -> Gain6/1
  Gain1/1 -> Add6/2
  Add6/1 -> Gain/1
  Gain6/1 -> Add1/1
  Add1/1 -> Display2/1
  Constant4/1 -> Add1/2

== system singledof_base/AI DI/enc_slave ==
  Add1 : Sum
  Add6 : Sum
  Constant4 : Constant  Value=-19
  Display1 : Display
  Display2 : Display
  Display4 : Display
      settings: Decimation=200
  EL5101 Encoder : Subsystem  mask(EL5101){link_id=0}
      mask prompts: link_id "Link id (>=0)"
  EL5101 Latch : Subsystem  mask(EL5101){link_id=0}
      mask prompts: link_id "Link id (>=0)"
  Gain : Gain  Gain=1/(7500*4)
  Gain1 : Gain
  Gain6 : Gain  Gain=1/10*360
  Out1 : Outport
  wires:
  EL5101 Encoder/1(Out1) -> Display4/1, Add6/1, Out1/1
  EL5101 Latch/1(Out1) -> Display1/1, Gain1/1
  Gain/1 -> Gain6/1
  Gain1/1 -> Add6/2
  Add6/1 -> Gain/1
  Gain6/1 -> Add1/1
  Add1/1 -> Display2/1
  Constant4/1 -> Add1/2

== system singledof_base/AI DI/find_zero_during_init_m ==
  freeRun : Inport
  Clock : Clock
  Integer Delay : Delay  DelayLength=1
  Integer Delay1 : Delay  DelayLength=1
  Multiport Switch2 : MultiPortSwitch  DataPortOrder=Zero-based contiguous  Inputs=2  zeroidx=on
  and : Logic  DisableCoverage=on
  and1 : Logic  DisableCoverage=on  Operator=NOT
  max : RelationalOperator  DisableCoverage=on  Operator=<=
  max_val : Constant  DisableCoverage=on  Value=0.5
  min : RelationalOperator  DisableCoverage=on  Operator=<=
  min_val : Constant  DisableCoverage=on  Value=.2
  moving avg : Subsystem
  comp : Outport
  tag scope: settozero4=global
  wires:
  moving avg/1(avg) -> Multiport Switch2/3
  max/1 -> and/2, and1/1
  min/1 -> and/1
  max_val/1 -> max/2
  min_val/1 -> min/1
  Clock/1 -> min/2, max/1
  and/1 -> moving avg/2(active), Multiport Switch2/1
  Integer Delay1/1 -> comp/1
  freeRun/1 -> moving avg/1(force)
  Multiport Switch2/1 -> Integer Delay1/1, Integer Delay/1
  Integer Delay/1 -> Multiport Switch2/2
  and1/1 -> [settozero4]

== system singledof_base/AI DI/find_zero_during_init_s ==
  freeRun : Inport
  Clock : Clock
  Integer Delay : Delay  DelayLength=1
  Integer Delay1 : Delay  DelayLength=1
  Multiport Switch2 : MultiPortSwitch  DataPortOrder=Zero-based contiguous  Inputs=2  zeroidx=on
  and : Logic  DisableCoverage=on
  and1 : Logic  DisableCoverage=on  Operator=NOT
  max : RelationalOperator  DisableCoverage=on  Operator=<=
  max_val : Constant  DisableCoverage=on  Value=0.5
  min : RelationalOperator  DisableCoverage=on  Operator=<=
  min_val : Constant  DisableCoverage=on  Value=.2
  moving avg : Subsystem
  comp : Outport
  tag scope: settozero2=global
  wires:
  Integer Delay/1 -> Multiport Switch2/2
  Multiport Switch2/1 -> Integer Delay1/1, Integer Delay/1
  freeRun/1 -> moving avg/1(force)
  Integer Delay1/1 -> comp/1
  and/1 -> Multiport Switch2/1, moving avg/2(active)
  Clock/1 -> max/1, min/2
  min_val/1 -> min/1
  max_val/1 -> max/2
  min/1 -> and/1
  max/1 -> and/2, and1/1
  moving avg/1(avg) -> Multiport Switch2/3
  and1/1 -> [settozero2]

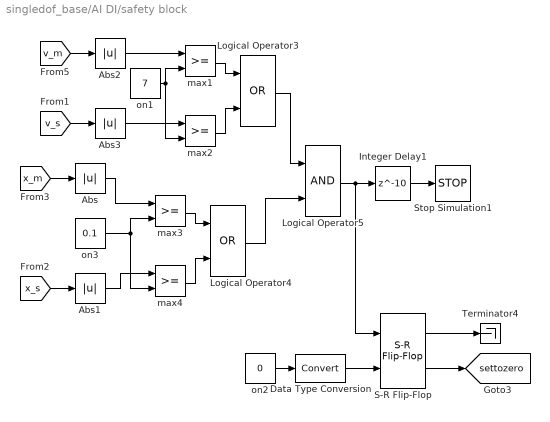
== system singledof_base/AI DI/safety block ==
  Abs{,1..3} (4 alike) : Abs
  Data Type Conversion : DataTypeConversion
  Integer Delay1 : Delay  DelayLength=10
  Logical Operator3 : Logic  Operator=OR  AllPortsSameDT=off  OutDataTypeStr=boolean
  Logical Operator4 : Logic  Operator=OR  AllPortsSameDT=off  OutDataTypeStr=boolean
  Logical Operator5 : Logic  AllPortsSameDT=off  OutDataTypeStr=boolean
  S-R Flip-Flop : simulink_extras/Flip Flops/S-R Flip-Flop  initial_condition=0
  Stop Simulation1 : Stop
  Terminator4 : Terminator
  max{1..4} (4 alike) : RelationalOperator  DisableCoverage=on
  on1 : Constant  DisableCoverage=on  Value=7
  on2 : Constant  DisableCoverage=on  Value=0
  on3 : Constant  DisableCoverage=on  Value=0.1
  tag scope: settozero=global
  wires:
  on1/1 -> max1/2, max2/2
  max1/1 -> Logical Operator3/1
  max2/1 -> Logical Operator3/2
  on2/1 -> Data Type Conversion/1
  Integer Delay1/1 -> Stop Simulation1/1
  S-R Flip-Flop/2 -> [settozero]
  Data Type Conversion/1 -> S-R Flip-Flop/2
  on3/1 -> max4/2, max3/2
  max3/1 -> Logical Operator4/1
  max4/1 -> Logical Operator4/2
  Abs/1 -> max3/1
  Abs1/1 -> max4/1
  Abs2/1 -> max1/1
  Abs3/1 -> max2/1
  Logical Operator3/1 -> Logical Operator5/1
  Logical Operator4/1 -> Logical Operator5/2
  Logical Operator5/1 -> Integer Delay1/1, S-R Flip-Flop/1
  S-R Flip-Flop/1 -> Terminator4/1
  [v_m] -> Abs2/1
  [v_s] -> Abs3/1
  [x_m] -> Abs/1
  [x_s] -> Abs1/1

== system singledof_base/AO DO/EL2008 DigitalOut ==
  In1 : Inport
  In2 : Inport  Port=2
  In3 : Inport  Port=3
  In4 : Inport  Port=4
  In5 : Inport  Port=5
  In6 : Inport  Port=6
  In7 : Inport  Port=7
  In8 : Inport  Port=8
  Mux : Mux  Inputs=8
  ec_EL2008_do : S-Function  FunctionName=ec_EL2008_do  Parameters=link_id  EnableBusSupport=off  mask{link_id=link_id}
      mask prompts: link_id "digital out id (start from 1)"
  wires:
  In8/1 -> Mux/8
  In7/1 -> Mux/7
  In6/1 -> Mux/6
  In5/1 -> Mux/5
  In4/1 -> Mux/4
  In3/1 -> Mux/3
  In2/1 -> Mux/2
  In1/1 -> Mux/1
  Mux/1 -> ec_EL2008_do/1

== system singledof_base/AO DO/EL4038 AnalogOut ==
  In1 : Inport
  In2 : Inport  Port=2
  In3 : Inport  Port=3
  In4 : Inport  Port=4
  In5 : Inport  Port=5
  In6 : Inport  Port=6
  In7 : Inport  Port=7
  In8 : Inport  Port=8
  Mux : Mux  Inputs=8
  ec_EL4038_dac : S-Function  FunctionName=ec_EL4038_dac  Parameters=link_id  EnableBusSupport=off  mask{link_id=link_id}
      mask prompts: link_id "analog out id (start from 1)"
  wires:
  In3/1 -> Mux/3
  In4/1 -> Mux/4
  In5/1 -> Mux/5
  In6/1 -> Mux/6
  In7/1 -> Mux/7
  In8/1 -> Mux/8
  In2/1 -> Mux/2
  In1/1 -> Mux/1
  Mux/1 -> ec_EL4038_dac/1

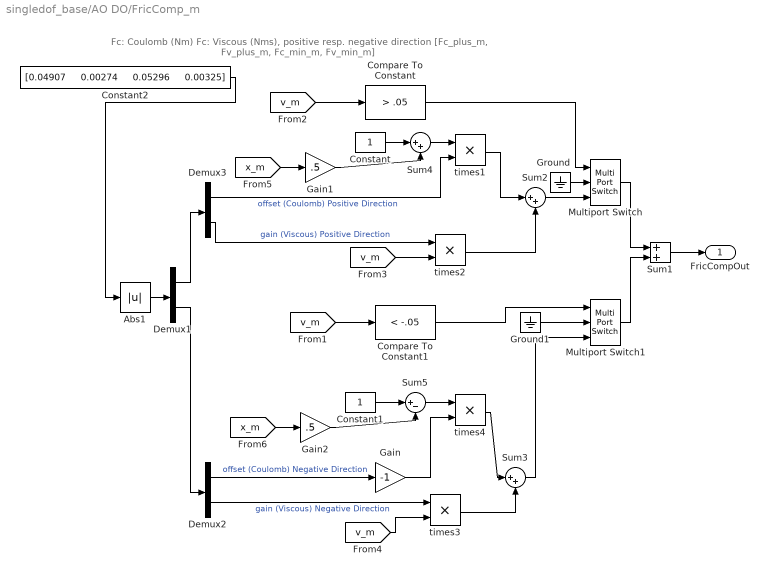
== system singledof_base/AO DO/FricComp_m ==
  note: Fc: Coulomb (Nm) Fc: Viscous (Nms), positive resp. negative direction [Fc_plus_m, Fv_plus_m, Fc_min_m, Fv_min_m]
  Abs1 : Abs
  Compare To Constant : simulink/Logic and Bit Operations/Compare To Constant  relop=>  const=.05  OutDataTypeStr=uint8
  Compare To Constant1 : simulink/Logic and Bit Operations/Compare To Constant  relop=<  const=-.05  OutDataTypeStr=uint8
  Constant : Constant
  Constant1 : Constant
  Constant2 : Constant  Value="[0.04907     0.00274     0.05296     0.00325]"
  Demux1 : Demux  Outputs=2
  Demux2 : Demux  Outputs=2
  Demux3 : Demux  Outputs=2
  Gain : Gain  Gain=-1
  Gain1 : Gain  Gain=.5
  Gain2 : Gain  Gain=.5
  Ground : Ground
  Ground1 : Ground
  Multiport Switch : MultiPortSwitch  DataPortOrder=Zero-based contiguous  Inputs=2  zeroidx=on
  Multiport Switch1 : MultiPortSwitch  DataPortOrder=Zero-based contiguous  Inputs=2  zeroidx=on
  Sum1 : Sum
  Sum2 : Sum  Inputs=|++
  Sum3 : Sum  Inputs=|++
  Sum4 : Sum  Inputs=|++
  Sum5 : Sum  Inputs=|+-
  times{1..4} (4 alike) : Product  Inputs=**
  FricCompOut : Outport
  wires:
  Abs1/1 -> Demux1/1
  Gain1/1 -> Sum4/2
  Constant/1 -> Sum4/1
  times4/1 -> Sum3/1
  Constant1/1 -> Sum5/1
  Sum5/1 -> times4/1
  Gain2/1 -> Sum5/2
  [x_m] -> Gain2/1
  times1/1 -> Sum2/1
  Sum4/1 -> times1/1
  [x_m] -> Gain1/1
  Gain/1 -> times4/2
  Multiport Switch1/1 -> Sum1/2
  Multiport Switch/1 -> Sum1/1
  Sum1/1 -> FricCompOut/1
  Sum3/1 -> Multiport Switch1/3
  Ground1/1 -> Multiport Switch1/2
  Compare To Constant1/1 -> Multiport Switch1/1
  [v_m] -> Compare To Constant1/1
  Ground/1 -> Multiport Switch/2
  times3/1 -> Sum3/2
  [v_m] -> times3/2
  Demux2/2 -> times3/1  "gain (Viscous) Negative Direction"
  Demux2/1 -> Gain/1  "offset (Coulomb) Negative Direction"
  Sum2/1 -> Multiport Switch/3
  times2/1 -> Sum2/2
  [v_m] -> times2/2
  Demux3/2 -> times2/1  "gain (Viscous) Positive Direction"
  Demux3/1 -> times1/2  "offset (Coulomb) Positive Direction"
  Demux1/1 -> Demux3/1
  Compare To Constant/1 -> Multiport Switch/1
  [v_m] -> Compare To Constant/1
  Demux1/2 -> Demux2/1
  Constant2/1 -> Abs1/1

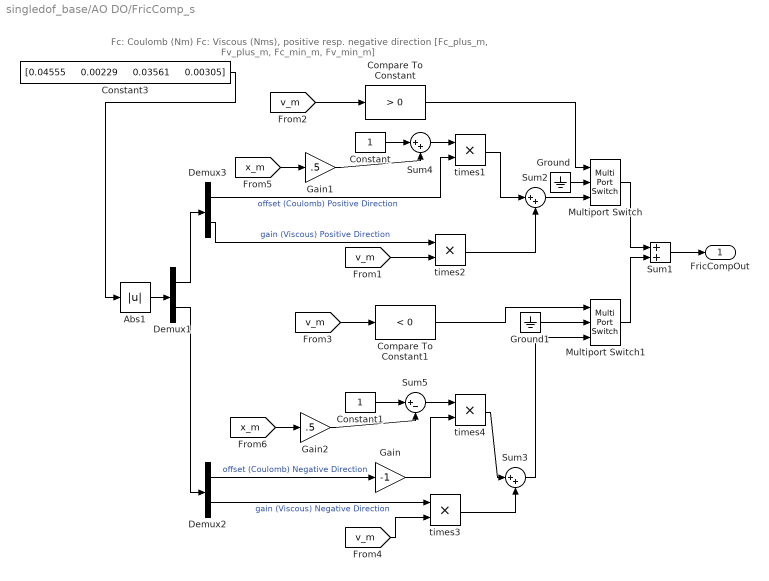
== system singledof_base/AO DO/FricComp_s ==
  note: Fc: Coulomb (Nm) Fc: Viscous (Nms), positive resp. negative direction [Fc_plus_m, Fv_plus_m, Fc_min_m, Fv_min_m]
  Abs1 : Abs
  Compare To Constant : simulink/Logic and Bit Operations/Compare To Constant  relop=>  const=0  OutDataTypeStr=uint8
  Compare To Constant1 : simulink/Logic and Bit Operations/Compare To Constant  relop=<  const=0  OutDataTypeStr=uint8
  Constant : Constant
  Constant1 : Constant
  Constant3 : Constant  Value="[0.04555     0.00229     0.03561     0.00305]"
  Demux1 : Demux  Outputs=2
  Demux2 : Demux  Outputs=2
  Demux3 : Demux  Outputs=2
  Gain : Gain  Gain=-1
  Gain1 : Gain  Gain=.5
  Gain2 : Gain  Gain=.5
  Ground : Ground
  Ground1 : Ground
  Multiport Switch : MultiPortSwitch  DataPortOrder=Zero-based contiguous  Inputs=2  zeroidx=on
  Multiport Switch1 : MultiPortSwitch  DataPortOrder=Zero-based contiguous  Inputs=2  zeroidx=on
  Sum1 : Sum
  Sum2 : Sum  Inputs=|++
  Sum3 : Sum  Inputs=|++
  Sum4 : Sum  Inputs=|++
  Sum5 : Sum  Inputs=|+-
  times{1..4} (4 alike) : Product  Inputs=**
  FricCompOut : Outport
  wires:
  Multiport Switch/1 -> Sum1/1
  Multiport Switch1/1 -> Sum1/2
  Constant3/1 -> Abs1/1
  Demux1/2 -> Demux2/1
  [v_m] -> Compare To Constant/1
  Compare To Constant/1 -> Multiport Switch/1
  Demux1/1 -> Demux3/1
  Demux3/1 -> times1/2  "offset (Coulomb) Positive Direction"
  Demux3/2 -> times2/1  "gain (Viscous) Positive Direction"
  [v_m] -> times2/2
  times2/1 -> Sum2/2
  Sum2/1 -> Multiport Switch/3
  Demux2/1 -> Gain/1  "offset (Coulomb) Negative Direction"
  Demux2/2 -> times3/1  "gain (Viscous) Negative Direction"
  [v_m] -> times3/2
  times3/1 -> Sum3/2
  Ground/1 -> Multiport Switch/2
  [v_m] -> Compare To Constant1/1
  Compare To Constant1/1 -> Multiport Switch1/1
  Ground1/1 -> Multiport Switch1/2
  Sum3/1 -> Multiport Switch1/3
  Sum1/1 -> FricCompOut/1
  Gain/1 -> times4/2
  [x_m] -> Gain1/1
  Sum4/1 -> times1/1
  times1/1 -> Sum2/1
  [x_m] -> Gain2/1
  Gain2/1 -> Sum5/2
  Sum5/1 -> times4/1
  Constant1/1 -> Sum5/1
  times4/1 -> Sum3/1
  Constant/1 -> Sum4/1
  Gain1/1 -> Sum4/2
  Abs1/1 -> Demux1/1

== system singledof_base/AO DO/LED ==
  note: groen slave
      | rood slave
      |
      | groen master
      | rood master
  Logical Operator{6,8..10} (4 alike) : Logic  Operator=OR  AllPortsSameDT=off  OutDataTypeStr=boolean
  Logical Operator11 : Logic  AllPortsSameDT=off  OutDataTypeStr=boolean
  Logical Operator2 : Logic  AllPortsSameDT=off  OutDataTypeStr=boolean
  Logical Operator7 : Logic  Operator=NOT  AllPortsSameDT=off  OutDataTypeStr=boolean
  Mux1 : Mux
  LED : Outport
  wires:
  [tau_dm_saturated] -> Logical Operator11/2
  Logical Operator11/1 -> Logical Operator8/2
  Logical Operator2/1 -> Logical Operator6/2
  [tau_rm_saturated] -> Logical Operator10/2
  [tau_rs_saturated] -> Logical Operator9/2
  Logical Operator10/1 -> Mux1/4
  Logical Operator9/1 -> Mux1/2
  Logical Operator8/1 -> Mux1/3
  Logical Operator7/1 -> Logical Operator10/1, Logical Operator8/1, Logical Operator9/1, Logical Operator6/1
  [init_complete] -> Logical Operator7/1
  Logical Operator6/1 -> Mux1/1
  [tau_ds_saturated] -> Logical Operator2/2
  [Passivity_enable] -> Logical Operator11/1, Logical Operator2/1
  Mux1/1 -> LED/1
